simulink model "Fig317"  (R2014b)
settings: Solver=ode3  StartTime=0.0  StopTime=5.24288  FixedStep=2e-6  RelTol=1e-5
libraries: commutil2 x1, commrandsrc2 x1
settings Model: Creator=Dennis Silage  LastModifiedBy=Silage
settings DataIOCC: SignalLoggingSaveFormat=ModelDataLogs
settings OptimizationCC: ExpressionDepthLimit=2147483647  InitFltsAndDblsToZero=on
settings DebuggingCC: UnderspecifiedInitializationDetection=Classic  MergeDetectMultiDrivingBlocksExec=none  SolverPrmCheckMsg=none  FcnCallInpInsideContextMsg=UseLocalSettings  StateNameClashWarn=warning
settings GRTTargetCC: CombineOutputUpdateFcns=off  GRTInterface=on

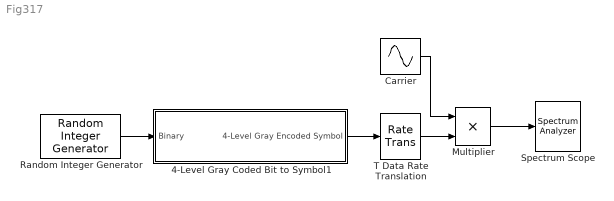
== system Fig317 ==
  4-Level Gray Coded Bit to Symbol1 : Subsystem
  Carrier : Sin  Amplitude=1.66666  Frequency=40000*pi  SampleTime=2e-6
  "Multiplier " : Product  RndMeth=Zero
  Random Integer Generator : commrandsrc2/Random Integer Generator  mul=2  seed=randseed  Ts=1e-3  frameBased=off  sampPerFrame=1  orient=off  outDataType=double
  Spectrum Scope : SpectrumAnalyzer
  T Data Rate Translation : RateTransition  OutPortSampleTime=2e-6
  wires:
  Random Integer Generator/1 -> 4-Level Gray Coded Bit to Symbol1/1(Binary)
  Carrier/1 -> "Multiplier "/1
  4-Level Gray Coded Bit to Symbol1/1(4-Level Gray Encoded Symbol) -> T Data Rate Translation/1
  T Data Rate Translation/1 -> "Multiplier "/2
  "Multiplier "/1 -> Spectrum Scope/1

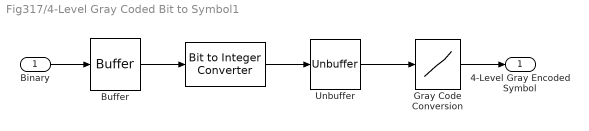
== system Fig317/4-Level Gray Coded Bit to Symbol1 ==
  Binary : Inport
  " " : commutil2/Bit to Integer Converter  nbits=2  bitOrder=MSB first  signedOutputValues=Unsigned  outDtype=Inherit via internal rule  outDtypeSigned=Inherit via internal rule
  Buffer : Buffer  N=2  TreatMby1Signals=One channel
  Gray Code Conversion : Lookup_n-D  NumberOfTableDimensions=1  BreakpointsForDimension1=[0, 1, 2, 3]  BreakpointsForDimension3=[5, 7]  BreakpointsForDimension1DataTypeStr=double  IndexSearchMethod=Linear search  Table=[0, 1, 3, 2]  TableDataTypeStr=double  InternalRulePriority=Speed  OutDataTypeStr=double  RndMeth=Simplest  InputSameDT=on
  Unbuffer : Unbuffer  SampleBasedProcessing=Same as frame based
  4-Level Gray Encoded Symbol : Outport
  wires:
  Gray Code Conversion/1 -> 4-Level Gray Encoded Symbol/1
  Binary/1 -> Buffer/1
  Buffer/1 -> " "/1
  " "/1 -> Unbuffer/1
  Unbuffer/1 -> Gray Code Conversion/1
